simulink model "prelab2018"  (R2018a)
settings: Solver=VariableStepAuto  StartTime=0.0  StopTime=2  RelTol=1e-3
undefined symbols (not defined in the file): A, A_d_hat, Ad_hat_10, Ad_hat_100, Ad_hat_20, Ad_hat_50, B, B_d_hat, Bd_hat_10, Bd_hat_100, Bd_hat_20, Bd_hat_50, C, K_d, K_d_10, K_d_20, K_d_50
settings Model: Creator=user  LastModifiedBy=armooga4
settings DataIOCC: ReturnWorkspaceOutputs=on
settings DebuggingCC: UnconnectedInputMsg=none  UnconnectedOutputMsg=none  UnconnectedLineMsg=none  SFMachineParentedDataDiag=error
settings SFSimCC: SimUseLocalCustomCode=on
settings RTWCC: RTWUseLocalCustomCode=on

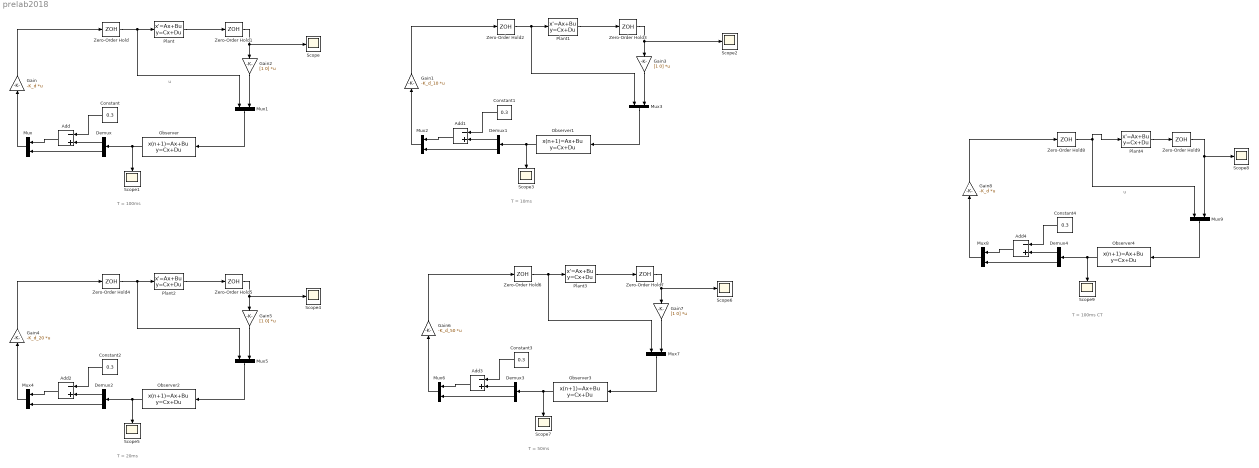
== system prelab2018 ==
  note: u
  note: T = 100ms
  note: T = 10ms
  note: T = 20ms
  note: T = 50ms
  note: u
  note: T = 100ms CT
  Add{,1..4} (5 alike) : Sum  Inputs=-+
  Constant{,1..4} (5 alike) : Constant  Value=0.3
  Demux{,1..4} (5 alike) : Demux  Outputs=2
  Gain : Gain  Gain=-K_d  Multiplication=Matrix(K*u)
  Gain1 : Gain  Gain=-K_d_10  Multiplication=Matrix(K*u)
  Gain{2..3,5,7} (4 alike) : Gain  Gain=[1 0]  Multiplication=Matrix(K*u)
  Gain4 : Gain  Gain=-K_d_20  Multiplication=Matrix(K*u)
  Gain6 : Gain  Gain=-K_d_50  Multiplication=Matrix(K*u)
  Gain8 : Gain  Gain=-K_d  Multiplication=Matrix(K*u)
  Mux{,1..9} (10 alike) : Mux  Inputs=2
  Observer : DiscreteStateSpace  A=Ad_hat_100  B=Bd_hat_100  C=eye(2)  D=[0 0;0 0]  SampleTime=0.1
  Observer1 : DiscreteStateSpace  A=Ad_hat_10  B=Bd_hat_10  C=eye(2)  D=[0 0;0 0]  SampleTime=-1
  Observer2 : DiscreteStateSpace  A=Ad_hat_20  B=Bd_hat_20  C=eye(2)  D=[0 0;0 0]  SampleTime=-1
  Observer3 : DiscreteStateSpace  A=Ad_hat_50  B=Bd_hat_50  C=eye(2)  D=[0 0;0 0]  SampleTime=-1
  Observer4 : DiscreteStateSpace  A=A_d_hat  B=B_d_hat  C=eye(2)  D=[0 0;0 0]  SampleTime=-1
  Plant{,1..3} (4 alike) : StateSpace  A=A  B=B  C=eye(2)  D=[0;0]  InitialCondition=0
  Plant4 : StateSpace  A=A  B=B  C=C  D=0  InitialCondition=0
  Scope{,1..9} (10 alike) : Scope
  Zero-Order Hold{,1,8..9} (4 alike) : ZeroOrderHold  SampleTime=0.1
  Zero-Order Hold2 : ZeroOrderHold  SampleTime=0.01
  Zero-Order Hold3 : ZeroOrderHold  SampleTime=0.01
  Zero-Order Hold4 : ZeroOrderHold  SampleTime=0.02
  Zero-Order Hold5 : ZeroOrderHold  SampleTime=0.02
  Zero-Order Hold6 : ZeroOrderHold  SampleTime=0.05
  Zero-Order Hold7 : ZeroOrderHold  SampleTime=0.05
  wires:
  Plant/1 -> Zero-Order Hold1/1
  Observer/1 -> Demux/1, Scope1/1
  Demux/2 -> Mux/2
  Demux/1 -> Add/2
  Mux/1 -> Gain/1
  Add/1 -> Mux/1
  Gain/1 -> Zero-Order Hold/1
  Constant/1 -> Add/1
  Zero-Order Hold/1 -> Plant/1, Mux1/1
  Mux1/1 -> Observer/1
  Gain2/1 -> Mux1/2
  Zero-Order Hold1/1 -> Scope/1, Gain2/1
  Gain3/1 -> Mux3/2
  Zero-Order Hold2/1 -> Plant1/1, Mux3/1
  Gain1/1 -> Zero-Order Hold2/1
  Zero-Order Hold3/1 -> Scope2/1, Gain3/1
  Demux1/1 -> Add1/2
  Plant1/1 -> Zero-Order Hold3/1
  Observer1/1 -> Demux1/1, Scope3/1
  Constant1/1 -> Add1/1
  Demux1/2 -> Mux2/2
  Add1/1 -> Mux2/1
  Mux2/1 -> Gain1/1
  Mux3/1 -> Observer1/1
  Gain5/1 -> Mux5/2
  Zero-Order Hold4/1 -> Plant2/1, Mux5/1
  Gain4/1 -> Zero-Order Hold4/1
  Zero-Order Hold5/1 -> Scope4/1, Gain5/1
  Demux2/1 -> Add2/2
  Plant2/1 -> Zero-Order Hold5/1
  Observer2/1 -> Demux2/1, Scope5/1
  Constant2/1 -> Add2/1
  Demux2/2 -> Mux4/2
  Add2/1 -> Mux4/1
  Mux4/1 -> Gain4/1
  Mux5/1 -> Observer2/1
  Add3/1 -> Mux6/1
  Constant3/1 -> Add3/1
  Plant3/1 -> Zero-Order Hold7/1
  Observer3/1 -> Demux3/1, Scope7/1
  Mux7/1 -> Observer3/1
  Demux3/2 -> Mux6/2
  Mux6/1 -> Gain6/1
  Zero-Order Hold7/1 -> Scope6/1, Gain7/1
  Gain6/1 -> Zero-Order Hold6/1
  Zero-Order Hold6/1 -> Plant3/1, Mux7/1
  Gain7/1 -> Mux7/2
  Demux3/1 -> Add3/2
  Zero-Order Hold9/1 -> Mux9/2, Scope8/1
  Demux4/1 -> Add4/2
  Demux4/2 -> Mux8/2
  Zero-Order Hold8/1 -> Plant4/1, Mux9/1
  Mux9/1 -> Observer4/1
  Add4/1 -> Mux8/1
  Plant4/1 -> Zero-Order Hold9/1
  Observer4/1 -> Demux4/1, Scope9/1
  Constant4/1 -> Add4/1
  Mux8/1 -> Gain8/1
  Gain8/1 -> Zero-Order Hold8/1
